simulink model "RS232_noHFC_loopback_1P"  (Simulink 7.8)
settings: Solver=VariableStepDiscrete  StartTime=0.0  StopTime=Inf  FixedStep=Ts/4  RelTol=1e-3
PreLoadFcn:
  | clear all;
  | close all;
  | clc;
  | 
  | Ts = 1;          % clk (period)
StartFcn:
  | clc;
  | close all;
  | 
  | %
  | %   RS232 port initialization
  | %
  | PORTNAME = 'COM34';
  | fprintf('\nOpening RS232 port %s ...... ', PORTNAME);
  | s1 = serial(PORTNAME,'BaudRate',9600,'Parity','none','DataBits',8);
  | set(s1, 'FlowControl', 'none');
  | set(s1, 'InputBufferSize', 64);
  | set(s1, 'OutputBufferSize', 1);
  | fopen(s1);
  | fprintf('\nRS232 port %s activated\n', PORTNAME);
  | 
  | b2o_s1 = uint8(0);
  | d2o_s1 = uint8(0);
  | b2r_s1 = uint8(0);
  | d2r_s1 = uint8(0);
  | rts_s1 = uint8(0);
  | cts_s1 = uint8(0);
StopFcn:
  | %
  | %   RS232 ports release
  | %
  | disp(' ');
  | disp('Deactivating RS232 port ......');
  | 
  | fclose(s1)
  | delete(s1)
  | clear s1
  | 
  | fprintf('RS232 port %s deactivated\n', PORTNAME);
libraries: simulink x1
settings Model: Creator=theodore  LastModifiedBy=theodore
settings DebuggingCC: SolverPrmCheckMsg=none
settings CodeAppCC: CustomSymbolStrType=$N$R$M_T

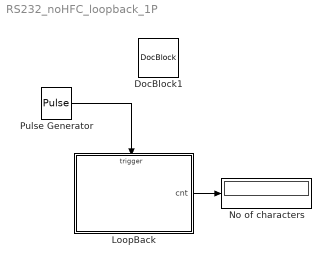
== system RS232_noHFC_loopback_1P ==
  DocBlock1 : simulink/Model-Wide Utilities/DocBlock  DocumentType=Text
  LoopBack : Stateflow chart  TreatAsAtomicUnit=on
  No of characters : Display
  Pulse Generator : DiscretePulseGenerator  PulseType=Time based  Period=Ts  PulseWidth=50
  wires:
  LoopBack/1(cnt) -> No of characters/1
  Pulse Generator/1 -> LoopBack/Trigger

== stateflow chart LoopBack ==
  state RxTxState
    en: ml('DIn_1');
    Val = ml.d2r_s1;
    ml.d2o_s1 = Val;
    ml('DOut_1');
    cnt = cnt + 1;
  state IniState
  IniState -> (junction 5) : {ml('B2O_1'); ml('B2R_1'); }
  (junction 5) -> RxTxState [order 2]
  (default) -> IniState : {cnt = 0;}
  (junction 5) -> IniState [order 1] : [ml.b2o_s1 > 0 ||  ml.b2r_s1 == 0 ]
  RxTxState -> IniState
  data: Val local double; cnt output double
  events: CLK input RISING_EDGE_EVENT
